simulink model "not_part_of_lab_03"  (R2024b)
settings: Solver=VariableStepAuto  StartTime=0.0  StopTime=10.0  RelTol=1e-3

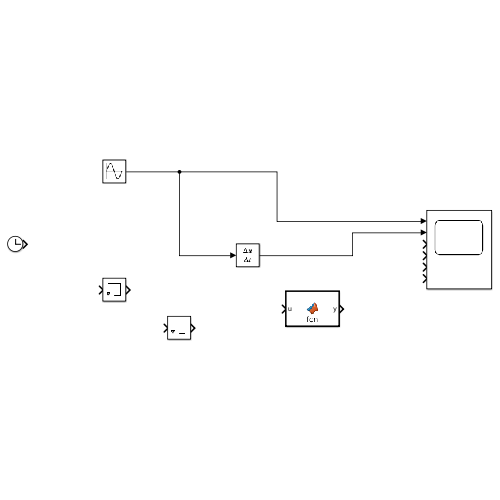
[thumbnail: Simulink's stored preview of the top-level diagram]
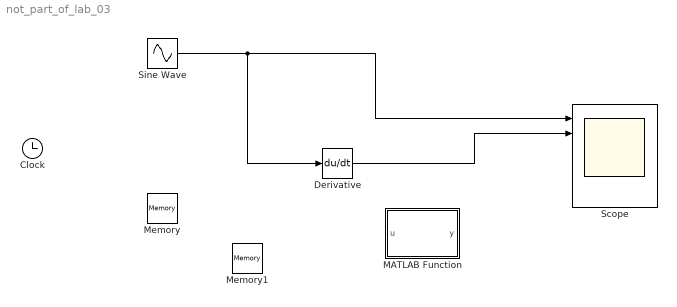
== system not_part_of_lab_03 ==
  Clock : Clock
  Derivative : Derivative
  MATLAB Function : MATLAB Function  TreatAsAtomicUnit=on
  Memory : Memory
  Memory1 : Memory
  Scope : Scope  NumInputPorts=6
  Sine Wave : Sin  SampleTime=0
  wires:
  Sine Wave/1 -> Derivative/1, Scope/1
  Derivative/1 -> Scope/2

== matlab function not_part_of_lab_03/MATLAB Function ==
  data: u input; y output
function y = fcn(u)

y = u;
